simulink model "sldemo_foreach_tiled"  (Simulink 7.6)
settings: Solver=FixedStepDiscrete  StartTime=0.0  StopTime=1.0  FixedStep=0.2  RelTol=1e-3
libraries: simulink x1
settings Model: Creator=The MathWorks Inc.
settings DataIOCC: SaveFormat=Structure
settings OptimizationCC: OptimizeModelRefInitCode=on  LifeSpan=1
settings RTWCC: SystemTargetFile=ert.tlc  TemplateMakefile=ert_default_tmf  Description=Real-Time Workshop Embedded Coder  GenerateReport=on  ProcessScript=ert_make_rtw_hook  IncludeHyperlinkInReport=on  LaunchReport=on
settings CodeAppCC: IgnoreCustomStorageClasses=off
settings ERTTargetCC: MultiwordLength=2048  GenerateSampleERTMain=on  MatFileLogging=on  SupportVariableSizeSignals=on  ERTCustomFileTemplate=example_file_process.tlc  ConvertIfToSwitch=off

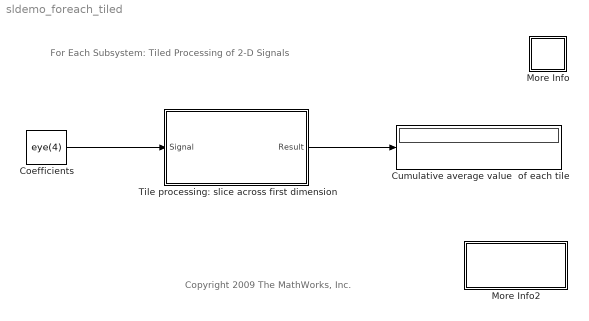
== system sldemo_foreach_tiled ==
  note: Copyright 2009 The MathWorks, Inc.
  note: For Each Subsystem:
      | Tiled Processing of 2-D Signals
  Coefficients : Constant  Value=eye(4)
  Cumulative average value  of each tile : Display
  More Info : Subsystem
      settings: OpenFcn=showdemo(bdroot(gcb))
      mask Display: disp('?')
  More Info2 : Subsystem
      settings: OpenFcn=sldemo_foreach_repeat_tile
      mask Display: disp('Double-Click for\nTile Repetition\nImplementation')
  Tile processing: slice across first dimension : Subsystem  TreatAsAtomicUnit=on
      settings: RTWFcnNameOpts=Use subsystem name  RTWFileNameOpts=Use function name
  wires:
  Coefficients/1 -> Tile processing: slice across first dimension/1(Signal)
  Tile processing: slice across first dimension/1(Result) -> Cumulative average value  of each tile/1

== system sldemo_foreach_tiled/More Info ==
  note: Bus Block Demonstration
  note: This demonstration shows how signals may be grouped and ungrouped while
      | retaining their names.  In this demonstration, 5 signals are created and labeled
      | appropriately.  These signals are then mux'd together to create a bus of signals.
      | This bus of signals is then fed into the Bus Selector block.  Inside of the Bus
      | Selector block, the Pulse and Chirp signals are chosen to be output from the
      | original signal bus.
      |
      | It is possible to place a nest signal buses and then still retrieve the original signal
      | with its label.

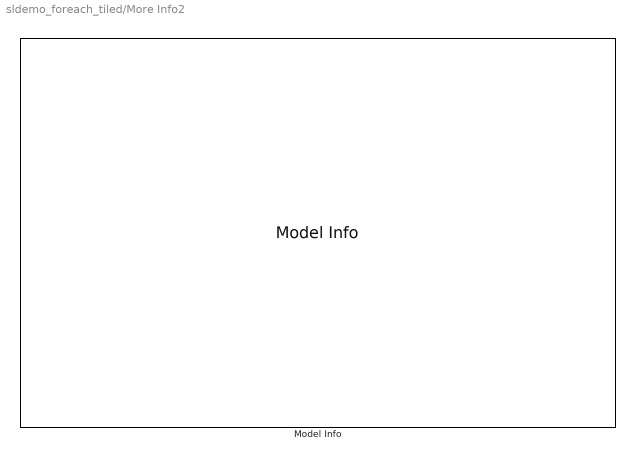
== system sldemo_foreach_tiled/More Info2 ==
  Model Info : simulink/Model-Wide Utilities/Model Info  SystemSampleTime=-1  InitialBlockCM=None  BlockCM=none  Frame=on  DisplayStringWithTags=Model Info  HorizontalTextAlignment=Left  LeftAlignmentValue=0.02  SourceBlockDiagram=sldemo_foreach_tiled  TagMaxNumber=20

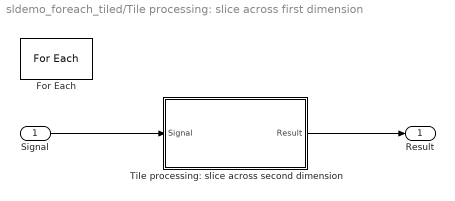
== system sldemo_foreach_tiled/Tile processing: slice across first dimension ==
  Signal : Inport  Partition=on  PartitionDimension=1  PartitionWidth=2
  For Each : ForEach  IndexMode=One-based
  Tile processing: slice across second dimension : Subsystem  TreatAsAtomicUnit=on
      settings: RTWFcnNameOpts=Use subsystem name  RTWFileNameOpts=Use function name
  Result : Outport  ConcatenationDimension=1
  wires:
  Signal/1 -> Tile processing: slice across second dimension/1(Signal)
  Tile processing: slice across second dimension/1(Result) -> Result/1

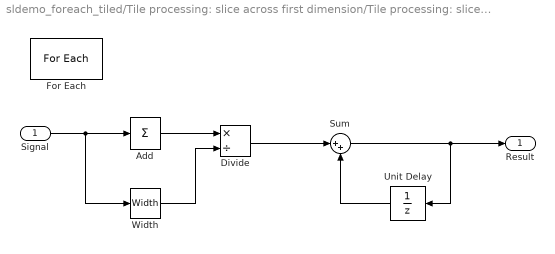
== system sldemo_foreach_tiled/Tile processing: slice across first dimension/Tile processing: slice across second dimension ==
  Signal : Inport  Partition=on  PartitionDimension=2  PartitionWidth=2
  Add : Sum  Inputs=+
  Divide : Product  Inputs=*/
  For Each : ForEach  IndexMode=One-based
  Sum : Sum  Inputs=|++
  Unit Delay : UnitDelay  SampleTime=-1
  Width : Width
  Result : Outport  ConcatenationDimension=2
  wires:
  Signal/1 -> Add/1, Width/1
  Add/1 -> Divide/1
  Width/1 -> Divide/2
  Divide/1 -> Sum/1
  Sum/1 -> Result/1, Unit Delay/1
  Unit Delay/1 -> Sum/2
